simulink model "MotorControl_HallSensor"  (R2018b)
settings: Solver=FixedStepDiscrete  StartTime=0.0  StopTime=10.0  FixedStep=1/5000  RelTol=1e-3  EnableMultiTasking=on
libraries: simulink x3, GPIO_Lib x2, ADC_Lib x1, STM32_Config_Lib x1, TIMERS_Lib x1
settings Model: Creator=Alex  LastModifiedBy=fenard1
settings DataIOCC: LimitDataPoints=on  SaveFormat=Array
settings OptimizationCC: DefaultParameterBehavior=Inlined  DefaultUnderspecifiedDataType=single  PassReuseOutputArgsAs=Individual arguments  ExpressionDepthLimit=2147483647  LifeSpan=1
settings DebuggingCC: UnderspecifiedInitializationDetection=Classic  MergeDetectMultiDrivingBlocksExec=none  SolverPrmCheckMsg=warning  UniqueDataStoreMsg=error  StateNameClashWarn=warning  StrictBusMsg=ErrorOnBusTreatedAsVector  SFUnexpectedBacktrackingDiag=warning  SFNoUnconditionalDefaultTransitionDiag=warning  SFUndirectedBroadcastEventsDiag=error  SFExecutionAtInitializationDiag=none
settings HardwareCC: ProdBitPerPointer=32  ProdBitPerSizeT=32  ProdBitPerPtrDiffT=32  ProdLargestAtomicInteger=Integer  ProdWordSize=32  ProdHWDeviceType=STMicroelectronics->STM32 32-bit Cortex-M  TargetLargestAtomicInteger=Integer  TargetLargestAtomicFloat=Float  TargetIntDivRoundTo=Zero  TargetEndianess=LittleEndian  TargetHWDeviceType=STMicroelectronics->STM32F4xx 32-bit Cortex-M4
settings ModelReferenceCC: PropagateSignalLabelsOutOfModel=off
settings SFSimCC: SimUseLocalCustomCode=off  CompileTimeRecursionLimit=0  EnableRuntimeRecursion=off  MATLABDynamicMemAlloc=off
settings RTWCC: SystemTargetFile=stm32.tlc  TemplateMakefile=stm32.tmf  Description=stm32 (Embedded Target)  GenerateReport=on  RTWUseLocalCustomCode=off  IncludeHyperlinkInReport=on
settings CodeAppCC: IgnoreCustomStorageClasses=off  IgnoreTestpoints=on  CustomSymbolStrType=$N$R$M  SimulinkBlockComments=off  InternalIdentifier=Classic
settings STFCustomTargetCC: TargetLangStandard=C99 (ISO)  CodeReplacementLibrary=ARM CMSIS SIN COS  ParMdlRefBuildCompliant=on  IncludeMdlTerminateFcn=off  CombineOutputUpdateFcns=on  ERTCustomFileBanners=on  SupportComplex=off  SupportContinuousTime=off  SupportNonInlinedSFcns=off  RemoveResetFunc=on  ParenthesesLevel=Maximum  CastingMode=Standards  MATLABClassNameForMDSCustomization=Simulink.SoftwareTarget.ERTCustomization  SystemTargetFile=stm32.tlc
settings ERTTargetCC: TargetLangStandard=C99 (ISO)  CodeReplacementLibrary=ARM CMSIS SIN COS  MultiwordLength=2048  CompOptLevelCompliant=off  ConcurrentExecutionCompliant=off  IncludeMdlTerminateFcn=off  SupportComplex=off  ParenthesesLevel=Maximum  CastingMode=Standards  ModelStepFunctionPrototypeControlCompliant=off  CPPClassGenCompliant=off  UseToolchainInfoCompliant=off  ERTSrcFileBannerTemplate=sourceFileTemplate.cgt  ERTHdrFileBannerTemplate=sourceFileTemplate.cgt  ERTDataSrcFileTemplate=sourceFileTemplate.cgt  ERTDataHdrFileTemplate=sourceFileTemplate.cgt  ERTCustomFileTemplate=customRoutineProcess.tlc  ConvertIfToSwitch=off  SuppressUnreachableDefaultCases=off  EnableSignedLeftShifts=off  EnableSignedRightShifts=off
settings ConfigComp: CovMetricSettings=dw  CovHtmlReporting=on  CovSaveCumulativeToWorkspaceVar=on  CovSaveSingleToWorkspaceVar=on  CovExternalEMLEnable=off  CovSFcnEnable=off

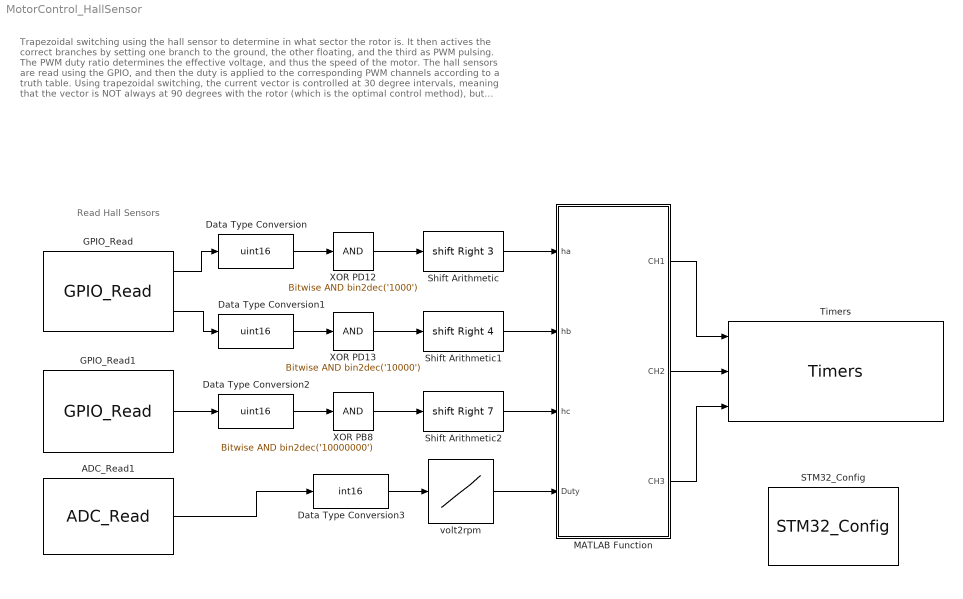
== system MotorControl_HallSensor ==
  note: Trapezoidal switching using the hall sensor to determine in what sector the rotor is. It then actives the correct branches by setting one branch to the ground, the other floating, and the third as PWM pulsing.
      |
      | The PWM duty ratio determines the effective voltage, and thus the speed of the motor. The hall sensors are read using the GPIO, and then the duty is applied to the corresponding PWM channels according to a truth table.
      |
      | Using trapezoidal switching, the current vector is controlled at 30 degree intervals, meaning that the vector is NOT always at 90 degrees with the rotor (which is the optimal control method), but rather oscillates with an error of +- 30 degrees. In this case, a ripple in the torque applied, and the motor produces extra noise, and consumes more current for the same mechanical power output (loss of efficiency)
      |
      | This Algorithm works in open loop (The motor speed is not measured)
  note: Read Hall Sensors
  ADC_Read1 : ADC_Lib/ADC_Read  ADC_Name=ADC1  ADC_Ch0=off  ADC_Ch1=off  ADC_Ch2=off  ADC_Ch3=off  ADC_Ch4=off  ADC_Ch5=off  ADC_Ch6=off  ADC_Ch7=off  ADC_Ch8=off  ADC_Ch9=off  ADC_Ch10=off  ADC_Ch11=on  ADC_Ch12=off  ADC_Ch13=off  ADC_Ch14=off  ADC_Ch15=off  ADC_Ch16=off  ADC_Ch17=off  ADC_Ch18=off  RgRk1=off  RgRk2=on  RgRk3=off  RgRk4=off  RgRk1_Ch=off  RgRk2_Ch=Ch11_r2  RgRk3_Ch=off  RgRk4_Ch=off  RgRk5=off  RgRk6=off  RgRk7=off  RgRk8=off  RgRk5_Ch=off  RgRk6_Ch=off  RgRk7_Ch=off  RgRk8_Ch=off  RgRk9=off  RgRk10=off  RgRk11=off  RgRk12=off  RgRk9_Ch=off  RgRk10_Ch=off  RgRk11_Ch=off  RgRk12_Ch=off  RgRk13=off  RgRk14=off  RgRk15=off  RgRk16=off  RgRk13_Ch=off  RgRk14_Ch=off  RgRk15_Ch=off  RgRk16_Ch=off  InjRk1=off  InjRk2=off  InjRk3=off  InjRk4=off  InjRk1_Ch=off  InjRk2_Ch=off  InjRk3_Ch=off  InjRk4_Ch=off  ADC_Trig=T8_TRGO  ADC_TrigEdge=RISING  DmaReq=on  DMA_Buffer=128  ItReq=off  AWD_Mode=NOT_USED  AWD_Ch=0  AWD_HThres=0  AWD_LThres=0  AWD_En_Int=off  AWD2_HThres=0  AWD2_LThres=0  AWD2_En_Int=off  AWD3_HThres=0  AWD3_LThres=0  AWD3_En_Int=off  EOC_SEQ=on  EOC_IT=off  JEOC_IT=off  AWD_IT=off  OVR_IT=off  CpltTrans=off  HalfTrans=off  ADC_RegNb=2  ADC_RegCh0=off  ADC_RegCh1=off  ADC_RegCh2=off  ADC_RegCh3=off  ADC_RegCh4=off  ADC_RegCh5=off  ADC_RegCh6=off  ADC_RegCh7=off  ADC_RegCh8=off  ADC_RegCh9=off  ADC_RegCh10=off  ADC_RegCh11=on  ADC_RegCh12=off  ADC_RegCh13=off  ADC_RegCh14=off  ADC_RegCh15=off  ADC_RegCh16=off  ADC_RegCh17=off  ADC_RegCh18=off  ADC_InjNb=0  ADC_InjCh0=off  ADC_InjCh1=off  ADC_InjCh2=off  ADC_InjCh3=off  ADC_InjCh4=off  ADC_InjCh5=off  ADC_InjCh6=off  ADC_InjCh7=off  ADC_InjCh8=off  ADC_InjCh9=off  ADC_InjCh10=off  ADC_InjCh11=off  ADC_InjCh12=off  ADC_InjCh13=off  ADC_InjCh14=off  ADC_InjCh15=off  ADC_InjCh16=off  ADC_InjCh17=off  ADC_InjCh18=off  NbADC=1  CurrentADC=ADC1
      settings: SourceProductName=Target Support Package - STM32 Adapter
  Data Type Conversion : DataTypeConversion  OutDataTypeStr=uint16
  Data Type Conversion1 : DataTypeConversion  OutDataTypeStr=uint16
  Data Type Conversion2 : DataTypeConversion  OutDataTypeStr=uint16
  Data Type Conversion3 : DataTypeConversion  OutDataTypeStr=int16
  GPIO_Read : GPIO_Lib/GPIO_Read  Port_name=GPIOD  Pin_0=off  Pin_1=off  Pin_2=off  Pin_3=off  Pin_4=off  Pin_5=off  Pin_6=off  Pin_7=off  Pin_8=off  Pin_9=off  Pin_10=off  Pin_11=off  Pin_12=on  Pin_13=on  Pin_14=off  Pin_15=off  PinList="GPIOB8GPIOD12  13"
      settings: SourceProductName=Target Support Package - STM32 Adapter
  GPIO_Read1 : GPIO_Lib/GPIO_Read  Port_name=GPIOB  Pin_0=off  Pin_1=off  Pin_2=off  Pin_3=off  Pin_4=off  Pin_5=off  Pin_6=off  Pin_7=off  Pin_8=on  Pin_9=off  Pin_10=off  Pin_11=off  Pin_12=off  Pin_13=off  Pin_14=off  Pin_15=off  PinList="GPIOB8GPIOD12  13"
      settings: SourceProductName=Target Support Package - STM32 Adapter
  MATLAB Function : MATLAB Function  TreatAsAtomicUnit=on  SystemSampleTime=1/5000
      settings: AttributesFormatString=SystemSampleTime=%<SystemSampleTime>
  STM32_Config : STM32_Config_Lib/STM32_Config  Priority=0  Project_Path=.\  Config_File=F407IGH6_Eval_HallSensor.ioc  MCU_Name=STM32F417IGHx
      settings: SourceProductName=Target Support Package - STM32 Adapter
  Shift Arithmetic : ArithShift  BitShiftNumber=3  BitShiftDirection=Right
  Shift Arithmetic1 : ArithShift  BitShiftNumber=4  BitShiftDirection=Right
  Shift Arithmetic2 : ArithShift  BitShiftNumber=7  BitShiftDirection=Right
  Timers : TIMERS_Lib/Timers  currentTIM=TIM8  TIM_Name=TIM8  sysUsingTimer=on  TIM_APBClock=168000000  TIM_Set_Clk=on  TIM_Prescaler=7  TIM_Clock=21000000.00  Variable_frequency=off  TIM_Set_OutFreq=on  TIM_ARR=525  Output_frequency=40000.00  Repetition_counter=0  TIM_Mode=Center_Aligned_2  TIM_DMA=none  TIM_IRQ=off  TIM_IRQ_ONLY=off  TIM_UP=off  TIM_TRG=off  TIM_COM=off  TIM_BRK=off  NbTIM=1  CH1_enable=on  CH1N_enable=on  CH1_type=Output_PWM  CH1_DMA=off  CH1_int=off  CH1_edge=Rising  CH1_div=1  CH1_variable_duty=on  CH1_set_pulse=on  CH1_output_duty=50  CH1_pulse=262  CH2_enable=on  CH2N_enable=on  CH2_type=Output_PWM  CH2_DMA=off  CH2_int=off  CH2_edge=Rising  CH2_div=1  CH2_variable_duty=on  CH2_set_pulse=on  CH2_output_duty=50  CH2_pulse=262  CH3_enable=on  CH3N_enable=on  CH3_type=Output_PWM  CH3_DMA=off  CH3_int=off  CH3_edge=Rising  CH3_div=1  CH3_variable_duty=on  CH3_set_pulse=on  CH3_output_duty=50  CH3_pulse=262  CH4_enable=off  CH4N_enable=off  CH4_type=Unknown  CH4_DMA=off  CH4_int=off  CH4_edge=Rising  CH4_div=1  CH4_variable_duty=off  CH4_set_pulse=off  CH4_output_duty=0.00  CH4_pulse=0
      settings: SourceProductName=Target Support Package - STM32 Adapter
  XOR PB8 : simulink/Logic and Bit Operations/Bitwise Operator  logicop=AND  UseBitMask=on  BitMask=bin2dec('10000000')  BitMaskRealWorld=Stored Integer
  XOR PD12 : simulink/Logic and Bit Operations/Bitwise Operator  logicop=AND  UseBitMask=on  BitMask=bin2dec('1000')  BitMaskRealWorld=Stored Integer
  XOR PD13 : simulink/Logic and Bit Operations/Bitwise Operator  logicop=AND  UseBitMask=on  BitMask=bin2dec('10000')  BitMaskRealWorld=Stored Integer
  volt2rpm : Lookup_n-D  NumberOfTableDimensions=1  BreakpointsForDimension1=[0:100]*(4095/101)  BreakpointsForDimension1Min=0  BreakpointsForDimension1Max=4095  UseOneInputPortForAllInputData=on  Table=[0:100]  ExtrapMethod=Clip  OutDataTypeStr=double  RndMeth=Simplest  InputSameDT=on
  wires:
  XOR PD12/1 -> Shift Arithmetic/1
  XOR PD13/1 -> Shift Arithmetic1/1
  XOR PB8/1 -> Shift Arithmetic2/1
  MATLAB Function/2(CH2) -> Timers/2
  MATLAB Function/1(CH1) -> Timers/1
  MATLAB Function/3(CH3) -> Timers/3
  Shift Arithmetic1/1 -> MATLAB Function/2(hb)
  volt2rpm/1 -> MATLAB Function/4(Duty)
  Shift Arithmetic/1 -> MATLAB Function/1(ha)
  Shift Arithmetic2/1 -> MATLAB Function/3(hc)
  GPIO_Read1/1 -> Data Type Conversion2/1
  GPIO_Read/1 -> Data Type Conversion/1
  GPIO_Read/2 -> Data Type Conversion1/1
  Data Type Conversion3/1 -> volt2rpm/1
  Data Type Conversion/1 -> XOR PD12/1
  Data Type Conversion1/1 -> XOR PD13/1
  Data Type Conversion2/1 -> XOR PB8/1
  ADC_Read1/1 -> Data Type Conversion3/1

== matlab function MotorControl_HallSensor/MATLAB Function ==
  data: ha input; hb input; hc input; CH1 output; CH2 output; CH3 output; Duty input
function [CH1,CH2,CH3]=Hall_State(ha,hb,hc,Duty)

bc = ha & hb & ~hc;
ba = ~ha & hb & ~hc;
ca = ~ha & hb & hc;
cb = ~ha & ~hb & hc;
ab = ha & ~hb & hc;
ac = ha & ~hb & ~hc;

if bc
    CH1 = (-1);
    CH2 = (Duty);
    CH3 = (0);
elseif ba
    CH1 = (0);
    CH2 = (Duty);
    CH3 = (-1);
elseif ca
    CH1 = (0);
    CH2 = (-1);
    CH3 = (Duty);
elseif cb
    CH1 = (-1);
    CH2 = (0);
    CH3 = (Duty);
elseif ab
    CH1 = (Duty);
    CH2 = (0);
    CH3 = (-1);
elseif ac
    CH1 = (Duty);
    CH2 = (-1);
    CH3 = (0);
else
    CH1 = (-1);
    CH2 = (-1);
    CH3 = (-1);
end
